simulink model "prova_2019a"  (R2019a)
settings: Solver=ode45  StartTime=0.0  StopTime=0.7  FixedStep=0.01  RelTol=1e-3
values from neighbouring files (symbols this model uses):
  b_ck = 0.03    [Parameters.m]
  b_cv = 0.03    [Parameters.m]
  Jc = 0.01    [Parameters.m]
  Jeq = 0.5*(Je/(tauf)+M*Rw^2+4*Jw)    (= 39.7521)    [Parameters.m]
  k = 0.098    [Parameters.m]
  T_eq = -3970    [Parameters.m]
  v = (control.F(1))\(-control.U(:,:,1)*x_0 - control.K(1))    [Parameters.m]
  x_0 = [210;210;0]    [Parameters.m]
undefined symbols (not defined in the file or in its folder): T_l
settings Model: Creator=andre  LastModifiedBy=Federico Kieffer

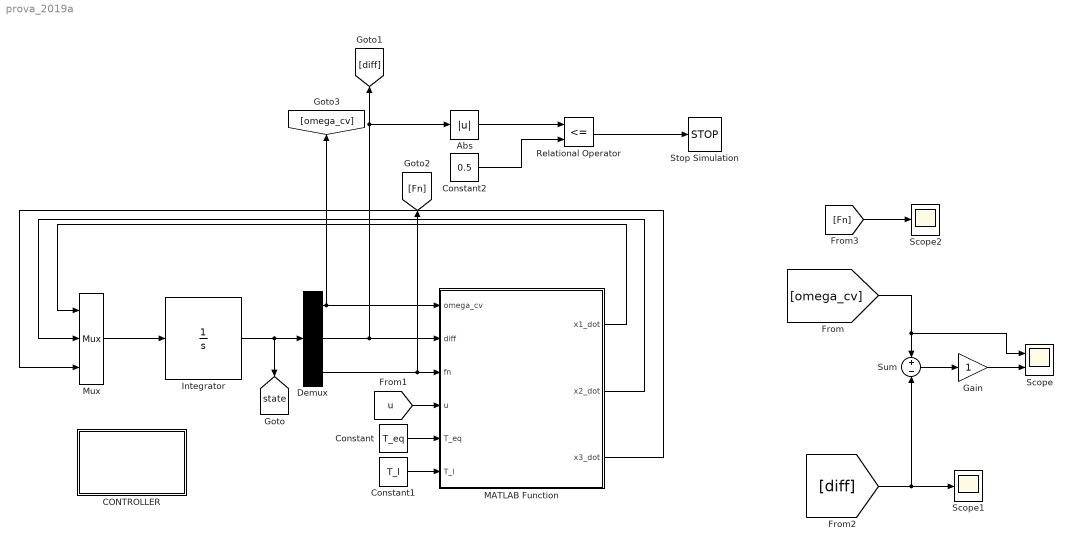
== system prova_2019a ==
  Abs : Abs
  CONTROLLER : Subsystem
  Constant : Constant  Value=T_eq
  Constant1 : Constant  Value=T_l
  Constant2 : Constant  Value=0.5
  Demux : Demux  Outputs=3
  Gain : Gain
  Integrator : Integrator  InitialCondition=x_0
  MATLAB Function : MATLAB Function  TreatAsAtomicUnit=on
  Mux : Mux  Inputs=3
  Relational Operator : RelationalOperator  Operator=<=  OutDataTypeStr=boolean  RndMeth=Simplest
  Scope : Scope  NumInputPorts=2
  Scope1 : Scope
  Scope2 : Scope
  Stop Simulation : Stop
  Sum : Sum  Inputs=+-
  tag scope: state=global
  wires:
  Mux/1 -> Integrator/1
  Integrator/1 -> Demux/1, [state]
  MATLAB Function/1(x1_dot) -> Mux/1
  MATLAB Function/2(x2_dot) -> Mux/2
  MATLAB Function/3(x3_dot) -> Mux/3
  Demux/2 -> MATLAB Function/2(diff), Abs/1, [diff]
  Demux/3 -> [Fn], MATLAB Function/3(fn)
  Constant/1 -> MATLAB Function/5(T_eq)
  Constant1/1 -> MATLAB Function/6(T_l)
  [u] -> MATLAB Function/4(u)
  Demux/1 -> MATLAB Function/1(omega_cv), [omega_cv]
  [Fn] -> Scope2/1
  [diff] -> Sum/2, Scope1/1
  [omega_cv] -> Scope/1, Sum/1
  Sum/1 -> Gain/1
  Gain/1 -> Scope/2
  Abs/1 -> Relational Operator/1
  Constant2/1 -> Relational Operator/2
  Relational Operator/1 -> Stop Simulation/1

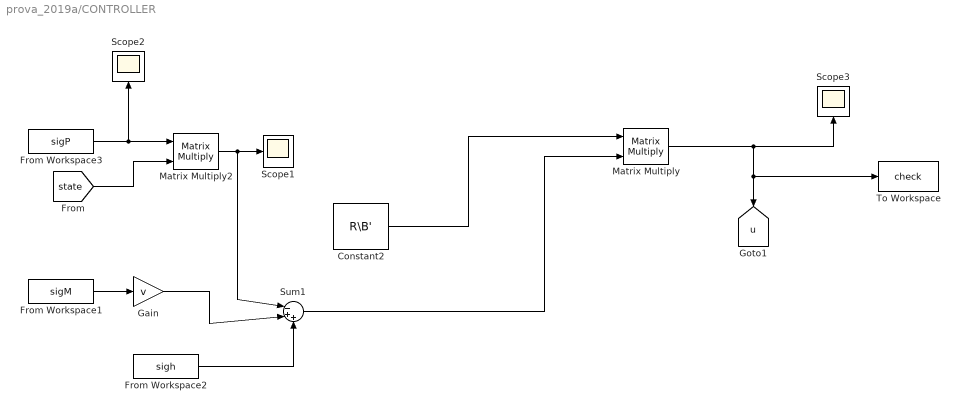
== system prova_2019a/CONTROLLER ==
  Constant2 : Constant  Value=R\B'  VectorParams1D=off
  From Workspace1 : FromWorkspace  VariableName=sigM  SampleTime=0
  From Workspace2 : FromWorkspace  VariableName=sigh  SampleTime=0
  From Workspace3 : FromWorkspace  VariableName=sigP  SampleTime=0
  Gain : Gain  Gain=v
  Matrix Multiply : Product  Multiplication=Matrix(*)
  Matrix Multiply2 : Product  Multiplication=Matrix(*)
  Scope1 : Scope
  Scope2 : Scope
  Scope3 : Scope
  Sum1 : Sum  Inputs=|-++
  To Workspace : ToWorkspace  VariableName=check  SampleTime=-1
  tag scope: u=global
  wires:
  Matrix Multiply2/1 -> Sum1/1, Scope1/1
  Matrix Multiply/1 -> [u], To Workspace/1, Scope3/1
  Gain/1 -> Sum1/2
  From Workspace2/1 -> Sum1/3
  From Workspace1/1 -> Gain/1
  Sum1/1 -> Matrix Multiply/2
  Constant2/1 -> Matrix Multiply/1
  From Workspace3/1 -> Matrix Multiply2/1, Scope2/1
  [state] -> Matrix Multiply2/2

== matlab function prova_2019a/MATLAB Function ==
  data: omega_cv input; x1_dot output; diff input; fn input; u input; T_eq input; T_l input; x2_dot output; Jeq parameter; Jc parameter; b_cv parameter; b_ck parameter; k parameter; x3_dot output
function [x1_dot,x2_dot,x3_dot] = dynamics(omega_cv,diff,fn,...
    u,T_eq,T_l,Jeq,Jc,b_cv, b_ck, k)

    x1 = omega_cv;
    x2 = diff;
    x3 = fn;
    %Jeq = 3;
    x1_dot = 1/Jeq*(-b_cv*x1 + T_eq - k*x3*sign(x2));
    x2_dot = (-b_cv/Jeq+b_ck/Jc)*x1 -(b_ck/Jc)*x2 -(k/Jeq+k/Jc)*x3*sign(x2)+...
        T_eq/Jeq %+ T_l/Jc; 
    x3_dot = u;
    
end
